simulink model "watertank_Comentado"  (R2025b)
settings: Solver=ode3  StartTime=0.0  StopTime=parInit.T_end  FixedStep=parSys.Ts  MaxStep=parSys.Ta  RelTol=1e-3  EnableMultiTasking=on
undefined symbols (not defined in the file): parSys, sigbuilder_block
libraries: simulink x3
settings Model: Creator=Wolfgang Kemmetmüller  LastModifiedBy=PC
settings SolverCC: AlgebraicLoopSolver=TrustRegion
settings DataIOCC: SaveFormat=Array  ReturnWorkspaceOutputs=off
settings OptimizationCC: ExpressionDepthLimit=2147483647.0  InitFltsAndDblsToZero=on  LifeSpan=inf
settings DebuggingCC: SaveWithParameterizedLinksMsg=none  UnderspecifiedInitializationDetection=Classic  MergeDetectMultiDrivingBlocksExec=none  SolverPrmCheckMsg=warning  MultiTaskDSMMsg=warning  MultiTaskCondExecSysMsg=none  UnconnectedInputMsg=warning  UnconnectedOutputMsg=warning  UnconnectedLineMsg=warning  StateNameClashWarn=warning  SFUnexpectedBacktrackingDiag=warning  SFNoUnconditionalDefaultTransitionDiag=warning  SFExecutionAtInitializationDiag=none  ArithmeticOperatorsInVariantConditions=warning
settings HardwareCC: ProdBitPerPointer=32.0  ProdBitPerSizeT=32.0  ProdBitPerPtrDiffT=32.0  ProdLargestAtomicFloat=None  ProdIntDivRoundTo=Undefined  ProdEndianess=Unspecified  ProdWordSize=32.0  ProdHWDeviceType=32-bit Generic
settings ModelReferenceCC: EnableRefExpFcnMdlSchedulingChecks=on  PropagateSignalLabelsOutOfModel=off
settings SFSimCC: SimUseLocalCustomCode=off  SimParseCustomCode=off  CustomCodeUndefinedFunction=UseInterfaceOnly
settings RTWCC: RTWUseLocalCustomCode=off  GPUComputeCapability=3.5  DLArmComputeVersion=19.05
settings CodeAppCC: StateflowObjectComments=on
settings GRTTargetCC: TargetLangStandard=C89/C90 (ANSI)  CombineOutputUpdateFcns=off  GRTInterface=on
settings ConfigComp: CovMetricSettings=dw  CovSaveCumulativeToWorkspaceVar=on  CovSaveSingleToWorkspaceVar=on  CovExternalEMLEnable=off  CovSFcnEnable=off

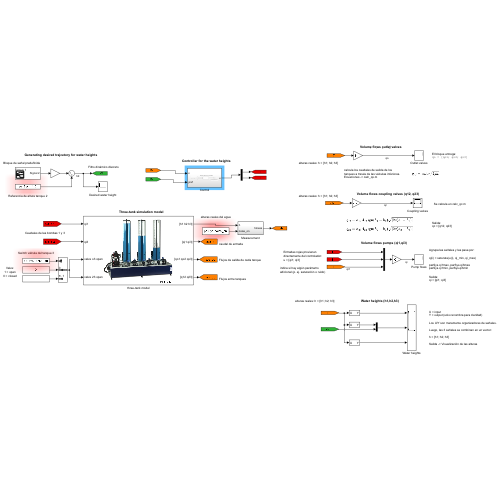
[thumbnail: Simulink's stored preview of the top-level diagram]
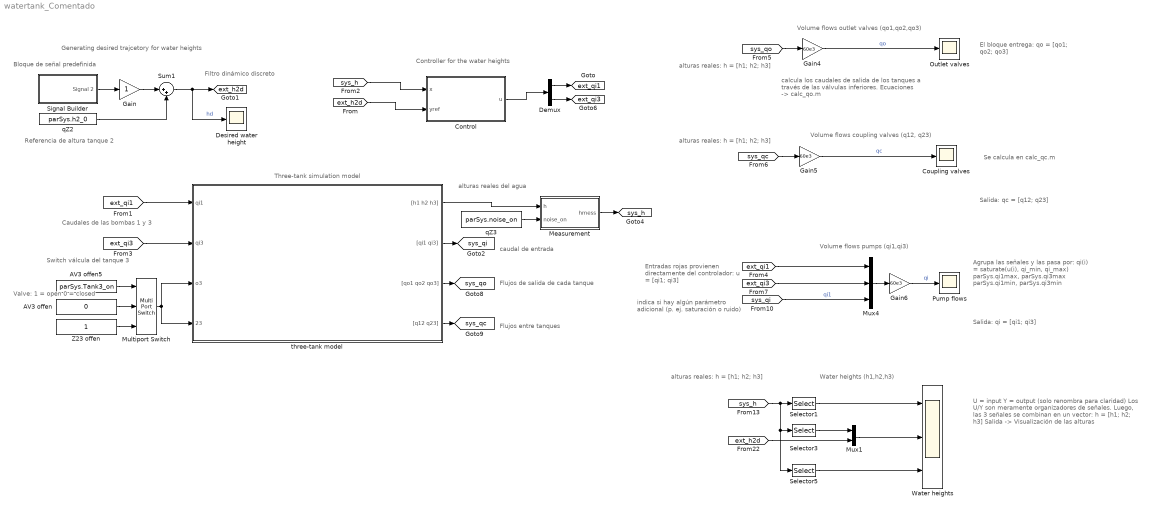
== system watertank_Comentado ==
  note: Referencia de altura tanque 2
  note: Generating desired trajcetory for water heights
  note: Valve:
      | 1 = open
      | 0 = closed
  note: Volume flows outlet valves (qo1,qo2,qo3)
  note: Water heights (h1,h2,h3)
  note: Volume flows coupling valves (q12, q23)
  note: Volume flows pumps (qi1,qi3)
  note: Controller for the water heights
  note: Three-tank simulation model
  note: Filtro dinámico discreto
  note: Caudales de las bombas 1 y 3
  note: Switch válcula del tanque 3
  note: alturas reales del agua
  note: caudal de entrada
  note: Flujos de salida de cada tanque
  note: Flujos entre tanques
  note: Bloque de señal predefinida
  note: calcula los caudales de salida de los
      | tanques a través de las válvulas inferiores.
      | Ecuaciones -> calc_qo.m
  note: alturas reales: h = [h1; h2; h3]
  note: El bloque entrega:
      | qo = [qo1; qo2; qo3]
  note: alturas reales: h = [h1; h2; h3]
  note: Se calcula en calc_qc.m
  note: Salida:
      | qc = [q12; q23]
  note: Entradas rojas provienen
      | directamente del controlador:
      | u = [qi1; qi3]
  note: indica si hay algún parámetro
      | adicional (p. ej. saturación o ruido)
  note: Agrupa las señales y las pasa por:
      |
      | qi(i) = saturate(u(i), qi_min, qi_max)
      |
      | parSys.qi1max, parSys.qi3max
      | parSys.qi1min, parSys.qi3min
  note: Salida:
      | qi = [qi1; qi3]
  note: alturas reales: h = [h1; h2; h3]
  note: U = input
      | Y = output (solo renombra para claridad)
      |
      | Los U/Y son meramente organizadores de señales.
      |
      | Luego, las 3 señales se combinan en un vector:
      |
      | h = [h1; h2; h3]
      |
      | Salida -> Visualización de las alturas
  AV3 offen : Constant  Value=0
  AV3 offen5 : Constant  Value=parSys.Tank3_on
  Control : Subsystem
  Coupling valves : Scope
      settings: ActiveDisplayYMinimum=-1.09509  ActiveDisplayYMaximum=1.61592  DataLoggingVariableName=ScopeData2
  Demux : Demux  Outputs=2
  Desired water height : Scope
      settings: TimeSpan=100  ActiveDisplayYMinimum=0.07884  ActiveDisplayYMaximum=0.29042
  Gain : Gain
  Gain4 : Gain  Gain=60e3
  Gain5 : Gain  Gain=60e3
  Gain6 : Gain  Gain=60e3
  Measurement : Subsystem
  Multiport Switch : MultiPortSwitch  DataPortOrder=Zero-based contiguous  Inputs=2  zeroidx=on  SaturateOnIntegerOverflow=off  InputSameDT=off
  Mux1 : Mux  Inputs=2
  Mux4 : Mux  Inputs=3
  Outlet valves : Scope
      settings: ActiveDisplayYMinimum=0.84233  ActiveDisplayYMaximum=1.52316  DataLoggingVariableName=ScopeData3
  Pump flows : Scope
      settings: ActiveDisplayYMinimum=-0.5625  ActiveDisplayYMaximum=5.0625  DataLoggingVariableName=ScopeData4
  Selector1 : Selector  InputPortWidth=3  IndexOptions=Index vector (dialog)  Indices=1  OutputSizes=1
  Selector3 : Selector  InputPortWidth=3  IndexOptions=Index vector (dialog)  Indices=2  OutputSizes=1
  Selector5 : Selector  InputPortWidth=3  IndexOptions=Index vector (dialog)  Indices=3  OutputSizes=1
  Signal Builder : Subsystem  Tag=STV Subsys  LoadFcn=sigbuilder_block('load');  StartFcn=sigbuilder_block('start');  StopFcn=sigbuilder_block('stop');  ClipboardFcn=sigbuilder_block('clipboard');  mask(Sigbuilder block){tuvar=[0:10]}
      mask help: Simulink:masks:SigbuilderBlock_MD
      mask init:
      | if ~strcmp(get_param(bdroot(gcbh),'SimulationStatus'),'stopped') tuvar = sigbuilder_block('maskInit'); end
      settings: CopyFcn=sigbuilder_block('copy');  DeleteFcn=sigbuilder_block('delete');  ModelCloseFcn=sigbuilder_block('modelClose');  PreSaveFcn=sigbuilder_block('preSave');  PauseFcn=sigbuilder_block('pause');  ContinueFcn=sigbuilder_block('continue');  NameChangeFcn=sigbuilder_block('namechange');  OpenFcn=sigbuilder_block('open',[316.5 171.75 805.5 485.25 ]);  CloseFcn=sigbuilder_block('close');
      mask Display: plot(0, 0, 100, 100,[2, 2, 32, 32, 2], [68, 8, 8, 68, 68],[32, 2], [38, 38], [32, 19, 2],[53, 60, 44], [32, 17, 17, 2],[16, 16, 31, 31]);txt = getActiveGroup(gcbh);text(2, 100, txt,'verticalAlignment', 'top');
  Sum1 : Sum  Inputs=|++
  Water heights : Scope  NumInputPorts=3
      settings: TimeSpan=1200  ActiveDisplayYMinimum=0.059987288353194321  ActiveDisplayYMaximum=0.7787974956664695  DataLoggingVariableName=ScopeData5
  Z23 offen : Constant
  qZ2 : Constant  Value=parSys.h2_0
  qZ3 : Constant  Value=parSys.noise_on
  three-tank model : Subsystem
      mask init:
      | S = get_param(gcb,'UserData');
      mask Display:
      | image(S.pic);
      | port_label('input', 1, 'qi1');
      | port_label('input', 2, 'qi3');
      | port_label('input', 3, 'valve o3 open');
      | port_label('input', 4, 'valve 23 open');
      | port_label('output', 1, '[h1 h2 h3]');
      | port_label('output', 2, '[qi1 qi3]');
      | port_label('output', 3, '[qo1 qo2 qo3]');
      | port_label('output', 4, '[q12 q23]');
  tag scope: ext_h2d=global, ext_qi1=global, ext_qi3=global, sys_h=global, sys_qc=global, sys_qi=global, sys_qo=global
  wires:
  Sum1/1 -> Desired water height/1, [ext_h2d]  "hd"
  qZ2/1 -> Sum1/2
  Demux/1 -> [ext_qi1]
  Demux/2 -> [ext_qi3]
  three-tank model/4("[q12 q23]") -> [sys_qc]
  three-tank model/3("[qo1 qo2 qo3]") -> [sys_qo]
  Z23 offen/1 -> Multiport Switch/3
  three-tank model/2("[qi1 qi3]") -> [sys_qi]
  three-tank model/1("[h1 h2 h3]") -> Measurement/1(h)
  AV3 offen5/1 -> Multiport Switch/1
  Measurement/1(hmess) -> [sys_h]
  [ext_qi1] -> three-tank model/1(qi1)
  Multiport Switch/1 -> three-tank model/3(o3), three-tank model/4(23)
  qZ3/1 -> Measurement/2(noise_on)
  AV3 offen/1 -> Multiport Switch/2
  [ext_qi3] -> three-tank model/2(qi3)
  Selector5/1 -> Water heights/3
  Mux4/1 -> Gain6/1
  Mux1/1 -> Water heights/2
  Selector1/1 -> Water heights/1
  Gain5/1 -> Coupling valves/1  "qc"
  Gain6/1 -> Pump flows/1  "qi"
  Selector3/1 -> Mux1/1
  [ext_h2d] -> Mux1/2
  [sys_qc] -> Gain5/1
  [sys_h] -> Selector5/1, Selector3/1, Selector1/1
  [sys_qo] -> Gain4/1
  Gain4/1 -> Outlet valves/1  "qo"
  [sys_qi] -> Mux4/3  "qi1"
  [ext_qi3] -> Mux4/2
  [ext_qi1] -> Mux4/1
  Gain/1 -> Sum1/1
  Signal Builder/1(Signal 2) -> Gain/1
  [sys_h] -> Control/1(x)
  [ext_h2d] -> Control/2(yref)
  Control/1(u) -> Demux/1

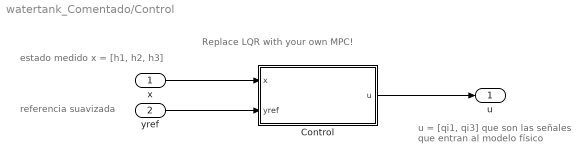
== system watertank_Comentado/Control ==
  note: estado medido x = [h1, h2, h3]
  note: Replace LQR with your own MPC!
  note: referencia suavizada
  note: u = [qi1, qi3] que son las señales
      | que entran al modelo físico
  x : Inport
  yref : Inport  Port=2
  Control : MATLAB Function  TreatAsAtomicUnit=on
  u : Outport
  wires:
  yref/1 -> Control/2(yref)
  x/1 -> Control/1(x)
  Control/1(u) -> u/1

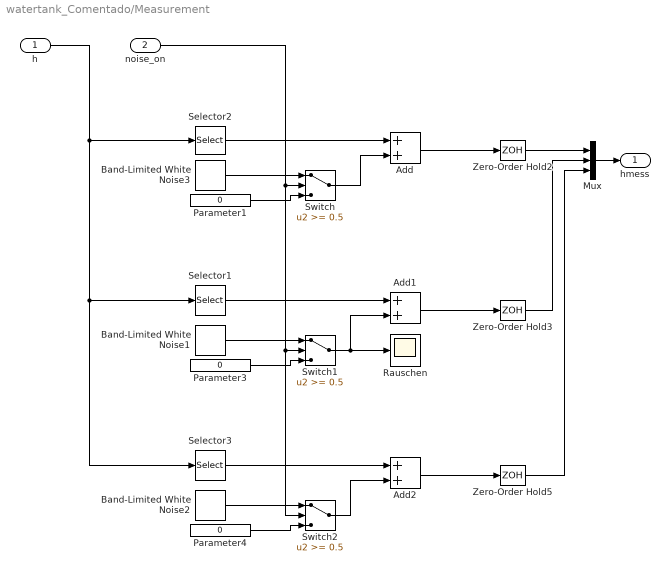
== system watertank_Comentado/Measurement ==
  h : Inport
  noise_on : Inport  Port=2
  Add : Sum
  Add1 : Sum
  Add2 : Sum
  Band-Limited White Noise1 : simulink/Sources/Band-Limited White Noise  Cov=parInit.meas.noisepow  Ts=parSys.Ts  seed=[981353]
  Band-Limited White Noise2 : simulink/Sources/Band-Limited White Noise  Cov=parInit.meas.noisepow  Ts=parSys.Ts  seed=[23343]
  Band-Limited White Noise3 : simulink/Sources/Band-Limited White Noise  Cov=parInit.meas.noisepow  Ts=parSys.Ts  seed=[23263]
  Mux : Mux  Inputs=3
  Parameter1 : Constant  Value=0  VectorParams1D=off
  Parameter3 : Constant  Value=0  VectorParams1D=off
  Parameter4 : Constant  Value=0  VectorParams1D=off
  Rauschen : Scope
      settings: TimeSpan=400  ActiveDisplayYMinimum=255  ActiveDisplayYMaximum=320  DataLoggingVariableName=ScopeData7
  Selector1 : Selector  InputPortWidth=3  IndexOptions=Index vector (dialog)  Indices=[2]  OutputSizes=1
  Selector2 : Selector  InputPortWidth=3  IndexOptions=Index vector (dialog)  Indices=[1]  OutputSizes=1
  Selector3 : Selector  InputPortWidth=3  IndexOptions=Index vector (dialog)  Indices=[3]  OutputSizes=1
  Switch : Switch  Threshold=0.5  SaturateOnIntegerOverflow=off  InputSameDT=off
  Switch1 : Switch  Threshold=0.5  SaturateOnIntegerOverflow=off  InputSameDT=off
  Switch2 : Switch  Threshold=0.5  SaturateOnIntegerOverflow=off  InputSameDT=off
  Zero-Order Hold2 : ZeroOrderHold  SampleTime=parSys.Ts
  Zero-Order Hold3 : ZeroOrderHold  SampleTime=parSys.Ts
  Zero-Order Hold5 : ZeroOrderHold  SampleTime=parSys.Ts
  hmess : Outport  VectorParamsAs1DForOutWhenUnconnected=off
  wires:
  Band-Limited White Noise3/1 -> Switch/1
  Switch/1 -> Add/2
  noise_on/1 -> Switch/2, Switch1/2, Switch2/2
  Selector2/1 -> Add/1
  Parameter1/1 -> Switch/3
  Band-Limited White Noise1/1 -> Switch1/1
  Switch1/1 -> Rauschen/1, Add1/2
  Selector1/1 -> Add1/1
  Parameter3/1 -> Switch1/3
  Band-Limited White Noise2/1 -> Switch2/1
  Switch2/1 -> Add2/2
  Parameter4/1 -> Switch2/3
  Add/1 -> Zero-Order Hold2/1
  Add1/1 -> Zero-Order Hold3/1
  Add2/1 -> Zero-Order Hold5/1
  Selector3/1 -> Add2/1
  h/1 -> Selector1/1, Selector3/1, Selector2/1
  Mux/1 -> hmess/1
  Zero-Order Hold2/1 -> Mux/1
  Zero-Order Hold3/1 -> Mux/2
  Zero-Order Hold5/1 -> Mux/3

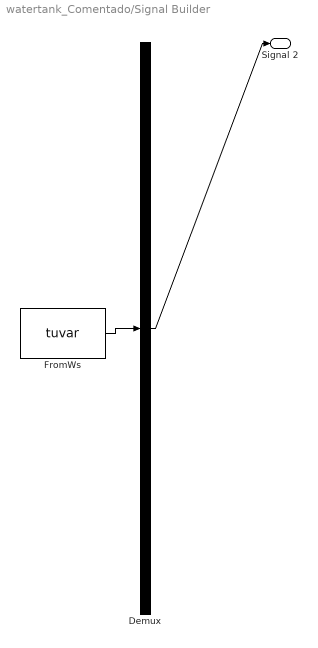
== system watertank_Comentado/Signal Builder ==
  Demux : Demux  Tag=STV Demux  Outputs=1
      settings: DisplayOption=none
  FromWs : FromWorkspace  Tag=STV FromWs  VariableName=tuvar
      SigBuilderData=|
      | common.afterFinalStr = 'Extrapolate'
      | common.sampleTime = 0
      | dataSet.timeRange = [0 1200]
      | dataSet.name = 'Group 1'
      | sbobj.Groups.Name = 'Group 1'
      | sbobj.Groups.Signals.Name = 'Signal 2'
      | sbobj.Groups.Signals.XData = [0 1 1 600 600 1200]
      | sbobj.Groups.Signals.YData = [0 0 0.1 0.1 0 0]
      | sbobj.Groups.TimeRange = [0 1200]
  Signal 2 : Outport  Tag=STV Outport  VectorParamsAs1DForOutWhenUnconnected=off
  wires:
  FromWs/1 -> Demux/1
  Demux/1 -> Signal 2/1

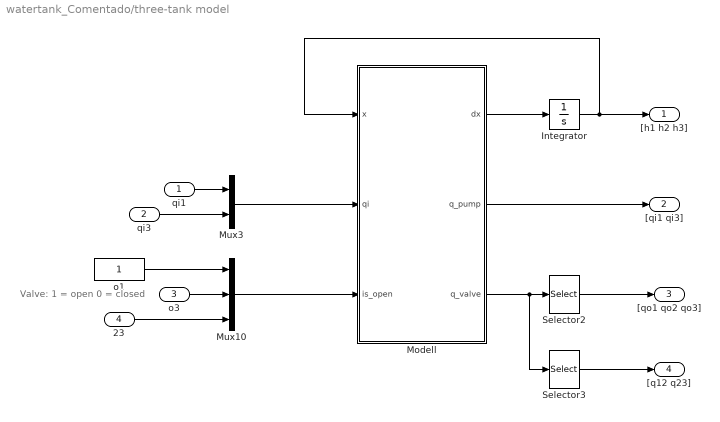
== system watertank_Comentado/three-tank model ==
  note: Valve:
      | 1 = open
      | 0 = closed
  qi1 : Inport
  qi3 : Inport  Port=2
  o3 : Inport  Port=3
  23 : Inport  Port=4
  Integrator : Integrator  InitialCondition=[parSys.h1_0; parSys.h2_0; parSys.h3_0]
  Modell : MATLAB Function  TreatAsAtomicUnit=on
  Mux10 : Mux  Inputs=3
  Mux3 : Mux  Inputs=2
  Selector2 : Selector  InputPortWidth=5  IndexOptions=Index vector (dialog)  Indices=[1 2 3]  OutputSizes=1
  Selector3 : Selector  InputPortWidth=5  IndexOptions=Index vector (dialog)  Indices=[4 5]  OutputSizes=1
  o1 : Constant
  "[h1 h2 h3]" : Outport  VectorParamsAs1DForOutWhenUnconnected=off
  "[qi1 qi3]" : Outport  Port=2  VectorParamsAs1DForOutWhenUnconnected=off
  "[qo1 qo2 qo3]" : Outport  Port=3  VectorParamsAs1DForOutWhenUnconnected=off
  "[q12 q23]" : Outport  Port=4  VectorParamsAs1DForOutWhenUnconnected=off
  wires:
  o1/1 -> Mux10/1
  qi1/1 -> Mux3/1
  qi3/1 -> Mux3/2
  Selector2/1 -> "[qo1 qo2 qo3]"/1
  Selector3/1 -> "[q12 q23]"/1
  23/1 -> Mux10/3
  o3/1 -> Mux10/2
  Mux10/1 -> Modell/3(is_open)
  Modell/1(dx) -> Integrator/1
  Integrator/1 -> Modell/1(x), "[h1 h2 h3]"/1
  Mux3/1 -> Modell/2(qi)
  Modell/3(q_valve) -> Selector3/1, Selector2/1
  Modell/2(q_pump) -> "[qi1 qi3]"/1

== matlab function watertank_Comentado/Control/Control ==
  settings: updateMethod=DISCRETE  sampleTime=parSys.Ts
  data: x input; u output; yref input
%Función para MPC

function u = fcn_MPC(x, yref)
% MPC simplificado para tanque 2

% Parámetros MPC simplificados (no se usan directamente)
N = 10;
Q = 10;
R = 1;

% Matrices discretas del sistema
Ad = parSys.Ad;
Bd = parSys.Bd;
Cd = parSys.Cd;

% Límite de la bomba 1
u_max = parSys.qi1max;

% Salida actual
y_actual = Cd * x;

% Error
error_y = yref - y_actual;

% Ganancia proporcional simulando el efecto MPC
Kp_mpc = 0.008;

% Control por feedback
u_feedback = Kp_mpc * error_y;

% Control feedforward (estado estacionario)
u_feedforward = parSys.uR(1);

% Entrada final bomba 1
u1 = u_feedforward + u_feedback;

% Saturación
u1 = max(0, min(u_max, u1));

% Bomba 3 fija en 0
u2 = 0;

u = [u1; u2];

end

== matlab function watertank_Comentado/three-tank model/Modell ==
  data: dx output; x input; qi input; is_open input; q_pump output; parSys parameter; q_valve output
function [dx, q_pump, q_valve] = fcn(x, qi, is_open, parSys)
%#codegen

[dx, q_pump, q_valve] = watertank_mfun(x, qi, is_open, parSys);

% Function end
end
